simulink model "WindEffectsModel"  (R2015b)
settings: Solver=VariableStepAuto  StartTime=0.0  StopTime=10.0  RelTol=1e-3
settings Model: Creator=jban039  LastModifiedBy=jeremie
settings ModelReferenceCC: ModelReferenceMinAlgLoopOccurrences=on

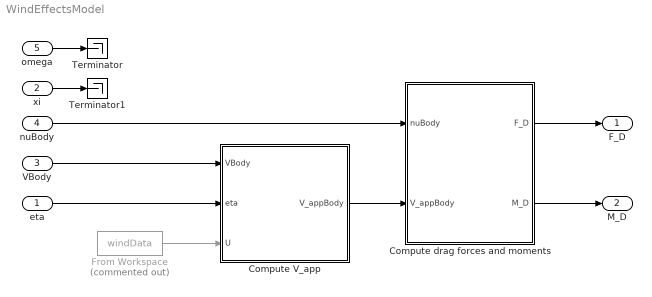
== system WindEffectsModel ==
  eta : Inport  PortDimensions=3
  xi : Inport  Port=2  PortDimensions=3
  VBody : Inport  Port=3  PortDimensions=3
  nuBody : Inport  Port=4  PortDimensions=3
  omega : Inport  Port=5  PortDimensions=Uav.N_ROTORS
  Compute V_app : MATLAB Function  TreatAsAtomicUnit=on
  Compute drag forces and moments : MATLAB Function  TreatAsAtomicUnit=on
  From Workspace : FromWorkspace  Commented=on  VariableName=windData  SampleTime=0
  Terminator : Terminator
  Terminator1 : Terminator
  F_D : Outport
  M_D : Outport  Port=2
  wires:
  Compute drag forces and moments/1(F_D) -> F_D/1
  Compute drag forces and moments/2(M_D) -> M_D/1
  Compute V_app/1(V_appBody) -> Compute drag forces and moments/2(V_appBody)
  omega/1 -> Terminator/1
  xi/1 -> Terminator1/1
  From Workspace/1 -> Compute V_app/3(U)
  nuBody/1 -> Compute drag forces and moments/1(nuBody)
  VBody/1 -> Compute V_app/1(VBody)
  eta/1 -> Compute V_app/2(eta)

== matlab function WindEffectsModel/Compute V_app ==
  data: VBody input; eta input; V_appBody output; U input size=3
function V_appBody = computeV_appBody(VBody, eta, U)
%#codegen

sPhi   = sin(eta(1));
sTheta = sin(eta(2));
sPsi   = sin(eta(3));
cPhi   = cos(eta(1));
cTheta = cos(eta(2));
cPsi   = cos(eta(3));

R = [cPsi*cTheta, cPsi*sTheta*sPhi-sPsi*cPhi, cPsi*sTheta*cPhi+sPsi*sPhi;
     sPsi*cTheta, sPsi*sTheta*sPhi+cPsi*cPhi, sPsi*sTheta*cPhi-cPsi*sPhi;
     -sTheta,     cTheta*sPhi,                cTheta*cPhi+sPsi*sPhi];

% Rotation matrix from Wind frame to Inertial frame 
R_U = [1, 0,  0;
       0, 1,  0;
       0, 0, -1];

V_appBody = VBody + R'*R_U*U;

== matlab function WindEffectsModel/Compute drag forces and moments ==
  data: nuBody input; V_appBody input; F_D output; M_D output; Uav parameter
function [F_D, M_D] = computeDrag(nuBody, V_appBody, Uav)
%#codegen

% Calculate drag force
F_D = 0.5 * Uav.RHO_AIR * Uav.C_D * (abs(V_appBody) .* V_appBody);

% Drag moment, applied to independent axes
M_D = 0.5 * Uav.RHO_AIR * Uav.C_DM * (abs(nuBody) .* nuBody);
